simulink model "Cascade_2"  (R2021a)
settings: Solver=FixedStepDiscrete  StartTime=0.0  StopTime=10.0  FixedStep=0.2  RelTol=1e-3
settings Model: Creator=Utkarsh Anand  LastModifiedBy=Utkarsh Anand
settings DataIOCC: SaveOutput=off  SaveTime=off

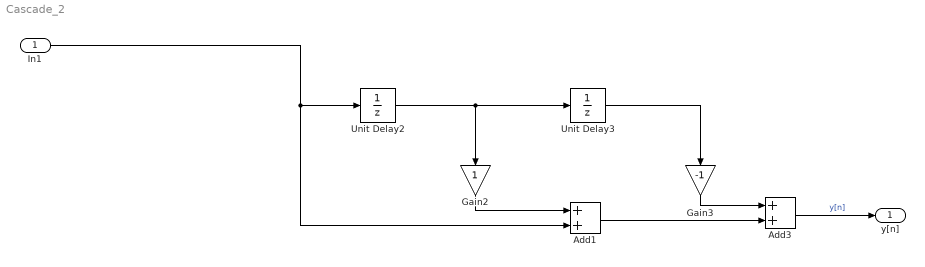
== system Cascade_2 ==
  In1 : Inport  OutDataTypeStr=double  PortDimensions=1  SampleTime=[0.20000000000000001,0]
  Add1 : Sum
  Add3 : Sum
  Gain2 : Gain
  Gain3 : Gain  Gain=-1
  Unit Delay2 : UnitDelay  SampleTime=-1  HasFrameUpgradeWarning=on
  Unit Delay3 : UnitDelay  SampleTime=-1  HasFrameUpgradeWarning=on
  y[n] : Outport  OutDataTypeStr=double  PortDimensions=1  SampleTime=[0.20000000000000001,0]
  wires:
  Unit Delay3/1 -> Gain3/1
  Add1/1 -> Add3/2
  Unit Delay2/1 -> Gain2/1, Unit Delay3/1
  Gain2/1 -> Add1/1
  Add3/1 -> y[n]/1  "y[n]"
  In1/1 -> Add1/2, Unit Delay2/1
  Gain3/1 -> Add3/1
